simulink model "iADC_gpioADCclk"  (Simulink 7.0)
settings: Solver=ode45  StartTime=0.0  StopTime=2000  RelTol=1e-3
libraries: xbsIndex_r4 x10, xps_library x6, casper_library x1
settings Model: Creator=user  LastModifiedBy=homin
settings DebuggingCC: SaveWithParameterizedLinksMsg=none

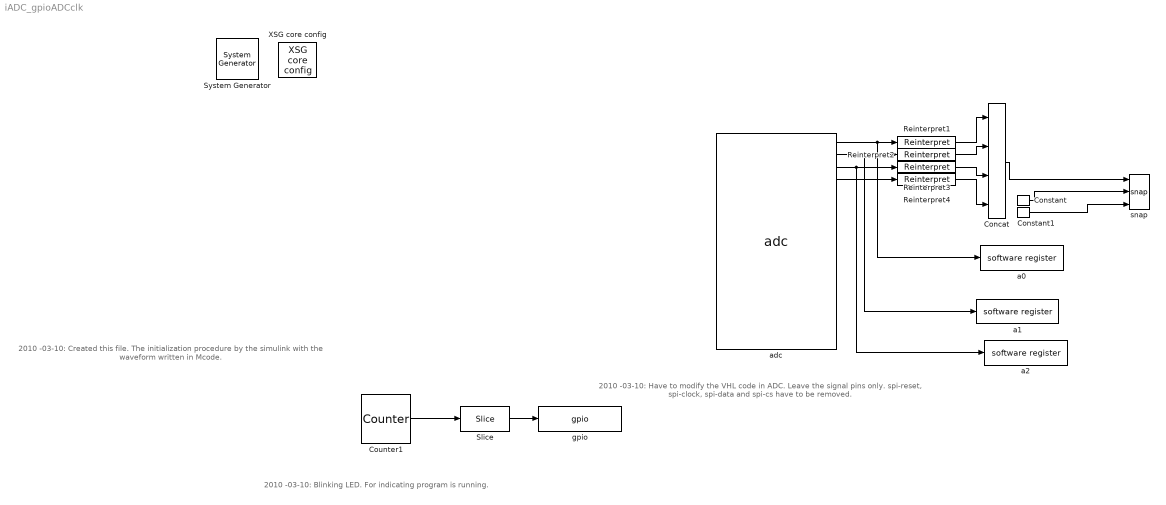
== system iADC_gpioADCclk ==
  note: 2010 -03-10:
      | Created this file. The initialization procedure by the simulink with
      | the waveform written in Mcode.
  note: 2010 -03-10:
      | Blinking LED. For indicating program is running.
  note: 2010 -03-10:
      | Have to modify the VHL code in ADC. Leave the signal pins only. spi-reset,
      | spi-clock, spi-data and spi-cs have to be removed.
  " System Generator" : xbsIndex_r4/ System Generator  Tag=genX  SystemSampleTime=-1  xilinxfamily=virtex5  part=xc5vsx95t  speed=-1  package=ff1136  synthesis_tool=XST  clock_wrapper=Clock Enables  directory=./iADC_gpioADCclk/sysgen  testbench=off  simulink_period=1  sysclk_period=5  dcm_input_clock_period=100  incr_netlist=off  trim_vbits=Everywhere in SubSystem  dbl_ovrd=According to Block Masks  core_generation=According to Block Masks  run_coregen=off  deprecated_control=off  eval_field=0  block_type=sysgen
      settings: block_version=10.1.3
  Concat : xbsIndex_r4/Concat  num_inputs=4  dbl_ovrd=off  block_type=concat
      settings: block_version=10.1.3
  Constant : xbsIndex_r4/Constant  arith_type=Boolean  const=0  n_bits=16  bin_pt=14  explicit_period=on  period=1  equ=P=C  opselect=C  inp2=PCIN>>17  opr=+  inp1=P  carry=CIN  dbl_ovrd=off  block_type=constant
  Constant1 : xbsIndex_r4/Constant  arith_type=Boolean  const=0  n_bits=16  bin_pt=14  explicit_period=on  period=1  equ=P=C  opselect=C  inp2=PCIN>>17  opr=+  inp1=P  carry=CIN  dbl_ovrd=off  block_type=constant
  Counter1 : xbsIndex_r4/Counter  cnt_type=Free Running  cnt_to=Inf  operation=Up  start_count=0  cnt_by_val=1  arith_type=Unsigned  n_bits=27  bin_pt=0  load_pin=off  rst=off  en=off  explicit_period=on  period=1  dbl_ovrd=off  use_behavioral_HDL=off  use_rpm=off  implementation=Fabric  block_type=counter
  Reinterpret{1..4} (4 alike) : xbsIndex_r4/Reinterpret  force_arith_type=on  arith_type=Unsigned  force_bin_pt=on  bin_pt=0  block_type=reinterpret
      settings: infoedit="Changes signal type without altering the binary representation.   You can changed the signal between signed and unsigned, and relocate the binary point.<P><P>Hardware notes: In hardware this block costs nothing.<P><P>Example:  Suppose the input is 6 bits wide, signed, with 2 fractional bits, and the output is forced to unsigned with 0 fractional bits.  Then an input of -2.0 (1110.00 in binary 2's complement) becomes an output of 56 (111000 in binary)."  block_version=10.1.3
  Slice : xbsIndex_r4/Slice  nbits=1  boolean_output=on  mode=Lower Bit Location + Width  bit1=27  base1=MSB of Input  bit0=26  base0=LSB of Input  dbl_ovrd=off  block_type=slice
      settings: infoedit="Extracts a given range of bits from each input sample and presents it at the output.  The output type is ordinarily unsigned with binary point at zero, but can be Boolean when the slice is one bit wide.<P><P>Hardware notes: In hardware this block costs nothing."  block_version=10.1.3
  XSG core config : xps_library/XSG core config  Tag=xps:xsg  SystemSampleTime=-1  hw_sys=ROACH:sx95t  ibob_linux=off  clk_src=adc0_clk  iBOB_clk_src=sys_clk  BEE2_ctrl_clk_src=sys_clk  BEE2_usr_clk_src=sys_clk  ROACH_clk_src=adc0_clk  CORR_clk_src=sys_clk  gpio_clk_io_group=iBOB:sma  gpio_clk_bit_index=0  clk_rate=200  sample_period=1  synthesis_tool=XST  mpc_type=powerpc440_ext
  a0 : xps_library/software register  Tag=xps:sw_reg  SystemSampleTime=-1  io_dir=To Processor  arith_type=Unsigned  bitwidth=32  bin_pt=0  sample_period=1  gw_name=iADC_gpioADCclk_a0_user_data_in
      link override convert: arith_type=Unsigned  n_bits=32  bin_pt=0
  a1 : xps_library/software register  Tag=xps:sw_reg  SystemSampleTime=-1  io_dir=To Processor  arith_type=Unsigned  bitwidth=32  bin_pt=0  sample_period=1  gw_name=iADC_gpioADCclk_a1_user_data_in
      link override convert: arith_type=Unsigned  n_bits=32  bin_pt=0
  a2 : xps_library/software register  Tag=xps:sw_reg  SystemSampleTime=-1  io_dir=To Processor  arith_type=Unsigned  bitwidth=32  bin_pt=0  sample_period=1  gw_name=iADC_gpioADCclk_a2_user_data_in
      link override convert: arith_type=Unsigned  n_bits=32  bin_pt=0
  adc : xps_library/adc  Tag=xps:adc  SystemSampleTime=-1  adc_brd=adc0  adc_clk_rate=800  adc_interleave=off  sample_period=1
  gpio : xps_library/gpio  Tag=xps:gpio  SystemSampleTime=-1  io_group=ROACH:led  io_dir=out  arith_type=Boolean  bitwidth=1  bin_pt=0  bit_index=1  sample_period=1  use_single_ended=off  use_ddr=off  reg_iob=on  reg_clk_phase=0  termination=None
      link override convert: arith_type=Boolean  n_bits=1  bin_pt=0
  snap : casper_library/Scopes/snap  SystemSampleTime=-1  nsamples=11
      link override addr/convert: arith_type=Unsigned  n_bits=32  bin_pt=0
      link override bram/convert_din: arith_type=Unsigned
      link override bram/iADC_gpioADCclk_snap_bram_data_out: arith_type=Unsigned
      link override bram/mem/sim_data_in: arith_type=Unsigned
      link override bram/tb_adc_5g_sysclk_snap_bram_data_out: arith_type=Unsigned
      link override ctrl/iADC_gpioADCclk_snap_ctrl_user_data_out: arith_type=Unsigned  n_bits=32  bin_pt=0  period=1
      link override ctrl/tb_adc_5g_sysclk_snap_ctrl_user_data_out: arith_type=Unsigned  n_bits=32  bin_pt=0  period=1
  wires:
  Counter1/1 -> Slice/1
  Slice/1 -> gpio/1
  Reinterpret1/1 -> Concat/1
  Reinterpret2/1 -> Concat/2
  Reinterpret3/1 -> Concat/3
  Reinterpret4/1 -> Concat/4
  Concat/1 -> snap/1
  Constant/1 -> snap/2
  Constant1/1 -> snap/3
  adc/1 -> Reinterpret1/1, a0/1
  adc/2 -> Reinterpret2/1, a1/1
  adc/3 -> Reinterpret3/1, a2/1
  adc/4 -> Reinterpret4/1
